simulink model "ThermalModel"  (R2018b)
settings: Solver=ode45  StartTime=0.0  StopTime=10.0  RelTol=1e-3  EnableMultiTasking=on
settings Model: Creator=sz609516  LastModifiedBy=fhu-eba
settings DataIOCC: LimitDataPoints=on  SaveFormat=Array  SignalLoggingSaveFormat=ModelDataLogs
settings OptimizationCC: ExpressionDepthLimit=2147483647  LifeSpan=inf
settings DebuggingCC: UnderspecifiedInitializationDetection=Classic  MergeDetectMultiDrivingBlocksExec=none  SolverPrmCheckMsg=warning  FcnCallInpInsideContextMsg=warning  StateNameClashWarn=warning  SFUnexpectedBacktrackingDiag=warning  SFNoUnconditionalDefaultTransitionDiag=warning
settings HardwareCC: ProdBitPerPointer=32  ProdBitPerSizeT=32  ProdBitPerPtrDiffT=32  ProdLargestAtomicFloat=None  ProdIntDivRoundTo=Undefined  ProdEndianess=Unspecified  ProdWordSize=32  ProdHWDeviceType=32-bit Generic
settings ModelReferenceCC: PropagateSignalLabelsOutOfModel=off
settings SFSimCC: SimUseLocalCustomCode=off
settings RTWCC: RTWUseLocalCustomCode=off
settings CodeAppCC: StateflowObjectComments=on
settings GRTTargetCC: TargetLangStandard=C89/C90 (ANSI)  GeneratePreprocessorConditionals=Disable all  CombineOutputUpdateFcns=off  GRTInterface=on
settings ConfigComp: CovMetricSettings=dw  CovHtmlReporting=on  CovSaveCumulativeToWorkspaceVar=on  CovSaveSingleToWorkspaceVar=on  CovExternalEMLEnable=off

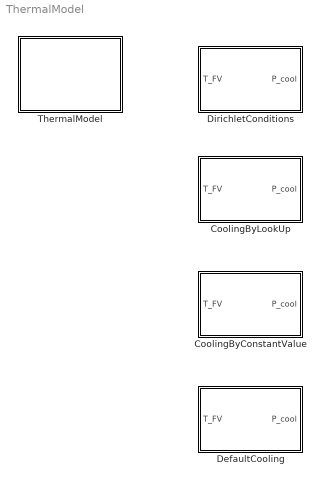
== system ThermalModel ==
  CoolingByConstantValue : Subsystem
  CoolingByLookUp : Subsystem
  DefaultCooling : Subsystem
  DirichletConditions : Subsystem
  ThermalModel : Subsystem

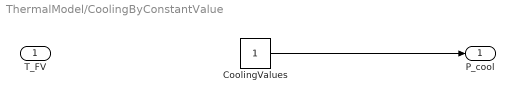
== system ThermalModel/CoolingByConstantValue ==
  T_FV : Inport
  CoolingValues : Constant
  P_cool : Outport
  wires:
  CoolingValues/1 -> P_cool/1

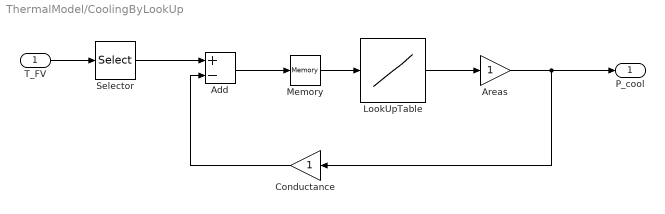
== system ThermalModel/CoolingByLookUp ==
  T_FV : Inport
  Add : Sum  Inputs=+-
  Areas : Gain
  Conductance : Gain
  LookUpTable : Lookup_n-D  NumberOfTableDimensions=1  BreakpointsForDimension1=[-5:5]  Table=tanh([-5:5])  ExtrapMethod=Clip  RndMeth=Simplest  InputSameDT=on
  Memory : Memory
  Selector : Selector  InputPortWidth=3  IndexOptions=Index vector (dialog)  Indices=[1 3]  OutputSizes=1
  P_cool : Outport
  wires:
  T_FV/1 -> Selector/1
  Selector/1 -> Add/1
  Add/1 -> Memory/1
  Conductance/1 -> Add/2
  Memory/1 -> LookUpTable/1
  LookUpTable/1 -> Areas/1
  Areas/1 -> Conductance/1, P_cool/1

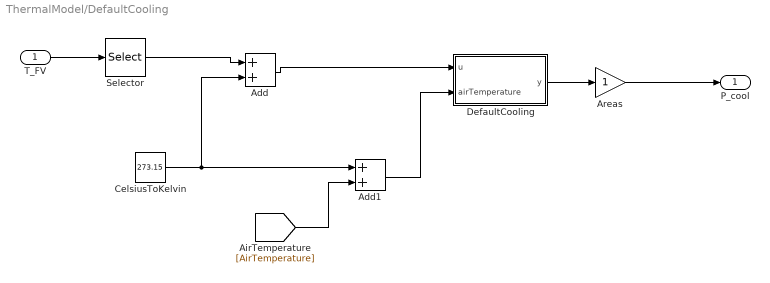
== system ThermalModel/DefaultCooling ==
  T_FV : Inport
  Add : Sum
  Add1 : Sum
  Areas : Gain
  CelsiusToKelvin : Constant  Value=273.15
  DefaultCooling : MATLAB Function  TreatAsAtomicUnit=on
  Selector : Selector  InputPortWidth=3  IndexOptions=Index vector (dialog)  Indices=[1 3]  OutputSizes=1
  P_cool : Outport
  wires:
  T_FV/1 -> Selector/1
  Selector/1 -> Add/1
  Add/1 -> DefaultCooling/1(u)
  DefaultCooling/1(y) -> Areas/1
  Areas/1 -> P_cool/1
  CelsiusToKelvin/1 -> Add1/1, Add/2
  Add1/1 -> DefaultCooling/2(airTemperature)
  [AirTemperature] -> Add1/2

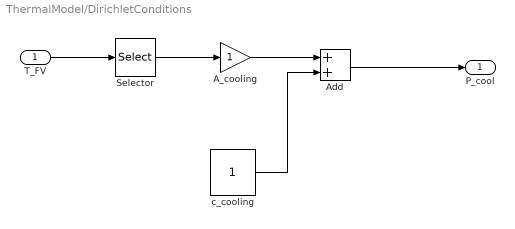
== system ThermalModel/DirichletConditions ==
  T_FV : Inport
  A_cooling : Gain
  Add : Sum
  Selector : Selector  InputPortWidth=3  IndexOptions=Index vector (dialog)  Indices=[1 3]  OutputSizes=1
  c_cooling : Constant
  P_cool : Outport
  wires:
  T_FV/1 -> Selector/1
  c_cooling/1 -> Add/2
  Add/1 -> P_cool/1
  Selector/1 -> A_cooling/1
  A_cooling/1 -> Add/1

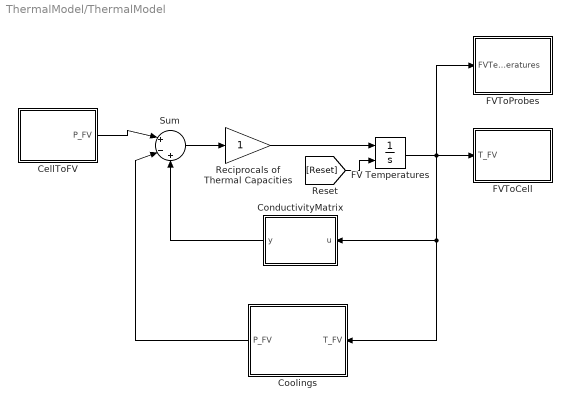
== system ThermalModel/ThermalModel ==
  CellToFV : Subsystem
  ConductivityMatrix : MATLAB Function  TreatAsAtomicUnit=on
  Coolings : Subsystem
  FV Temperatures : Integrator  ExternalReset=rising
  FVToCell : Subsystem
  FVToProbes : Subsystem
  Reciprocals of Thermal Capacities : Gain
  Sum : Sum  Inputs=|+-+
  wires:
  Sum/1 -> Reciprocals of Thermal Capacities/1
  Reciprocals of Thermal Capacities/1 -> FV Temperatures/1
  FV Temperatures/1 -> FVToProbes/1(FVTemperatures), FVToCell/1(T_FV), ConductivityMatrix/1(u), Coolings/1(T_FV)
  Coolings/1(P_FV) -> Sum/2
  CellToFV/1(P_FV) -> Sum/1
  ConductivityMatrix/1(y) -> Sum/3
  [Reset] -> FV Temperatures/2

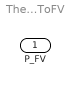
== system ThermalModel/ThermalModel/CellToFV ==
  P_FV : Outport

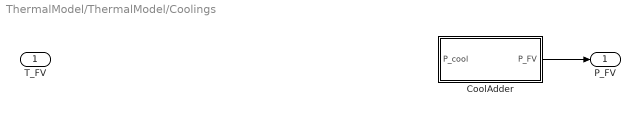
== system ThermalModel/ThermalModel/Coolings ==
  T_FV : Inport
  CoolAdder : Subsystem
  P_FV : Outport
  wires:
  CoolAdder/1(P_FV) -> P_FV/1

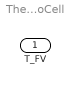
== system ThermalModel/ThermalModel/FVToCell ==
  T_FV : Inport

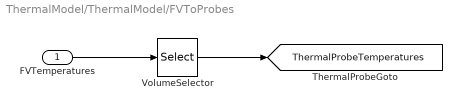
== system ThermalModel/ThermalModel/FVToProbes ==
  FVTemperatures : Inport
  VolumeSelector : Selector  InputPortWidth=3  IndexOptions=Index vector (dialog)  Indices=[1 3]  OutputSizes=1
  tag scope: ThermalProbeTemperatures=global
  wires:
  FVTemperatures/1 -> VolumeSelector/1
  VolumeSelector/1 -> [ThermalProbeTemperatures]

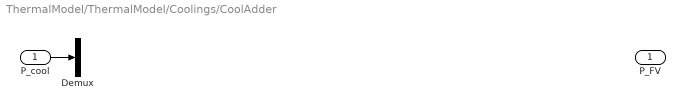
== system ThermalModel/ThermalModel/Coolings/CoolAdder ==
  P_cool : Inport
  Demux : Demux  Outputs=2
  P_FV : Outport
  wires:
  P_cool/1 -> Demux/1

== matlab function ThermalModel/DefaultCooling/DefaultCooling ==
  data: u input; y output; airTemperature input
function y = fcn(u, airTemperature)
    
y = DefaultCooling(u, airTemperature);

end

== matlab function ThermalModel/ConductivityMatrix ==
  data: u input; y output
function y = fcn(u)
    y = ConductivityMatrix(u);
end
